simulink model "ssc_lithium_cell_1RC"  (R2019b)
settings: Solver=ode15s  StartTime=0.0  StopTime=40000  MaxStep=60  RelTol=1e-3  EnableMultiTasking=on
PreLoadFcn:
  | ssc_lithium_cell_1RC_ini
undefined symbols (not defined in the file): Battery, sigbuilder_block
libraries: fl_lib x8, nesl_utility x6, ee_lib x1
Description:
  | Lithium Battery Cell - One RC-Branch Equivalent Circuit
  | 
  | This example shows how to model a lithium cell using the Simscape(TM)
  | language to implement the elements of an equivalent circuit model
  | with one RC branch. For the defining equations and their validation,
  | see T. Huria, M. Ceraolo, J. Gazzarri, R. Jackey. "High Fidelity Electrical
  | Model with Thermal Dependence for Characterization and Simulation of
  | High Power Lithium Battery Cells," IEEE International Electric Vehicle
  | Conference, March 2012.
  | 
  | A simple thermal model is used to model battery temperature. It is
  | assumed that cooling is primarily via convection, and that heating is
  | primarily from internal resistance. A battery pack can be modeled by
  | connecting multiple copies of the battery cell block in series.
  | 
  | 
  | 
  | Copyright 2008-2012 The MathWorks, Inc.
settings Model: Creator=MathWorks  LastModifiedBy=cpatel
settings DataIOCC: LimitDataPoints=on  SaveFormat=Array  SignalLoggingSaveFormat=ModelDataLogs  SaveOutput=off  SaveTime=off
settings OptimizationCC: ExpressionDepthLimit=2147483647  LifeSpan=inf
settings DebuggingCC: StateNameClashWarn=warning  SFUnexpectedBacktrackingDiag=warning  SFNoUnconditionalDefaultTransitionDiag=warning  SFExecutionAtInitializationDiag=none  ArithmeticOperatorsInVariantConditions=warning
settings HardwareCC: ProdBitPerPointer=32  ProdBitPerSizeT=32  ProdBitPerPtrDiffT=32  ProdLargestAtomicFloat=None  ProdIntDivRoundTo=Undefined  ProdEndianess=Unspecified  ProdWordSize=32  ProdHWDeviceType=32-bit Generic
settings ModelReferenceCC: PropagateSignalLabelsOutOfModel=off
settings SFSimCC: SimUseLocalCustomCode=off  CustomCodeUndefinedFunction=UseInterfaceOnly
settings RTWCC: RTWUseLocalCustomCode=off
settings CodeAppCC: StateflowObjectComments=on
settings GRTTargetCC: TargetLangStandard=C89/C90 (ANSI)  GeneratePreprocessorConditionals=Disable all  CombineOutputUpdateFcns=off  GRTInterface=on
settings ConfigComp: CovMetricSettings=dw  CovHtmlReporting=on  CovSaveCumulativeToWorkspaceVar=on  CovSaveSingleToWorkspaceVar=on  CovExternalEMLEnable=off
settings SimscapeCC: SimscapeNormalizeSystem=off

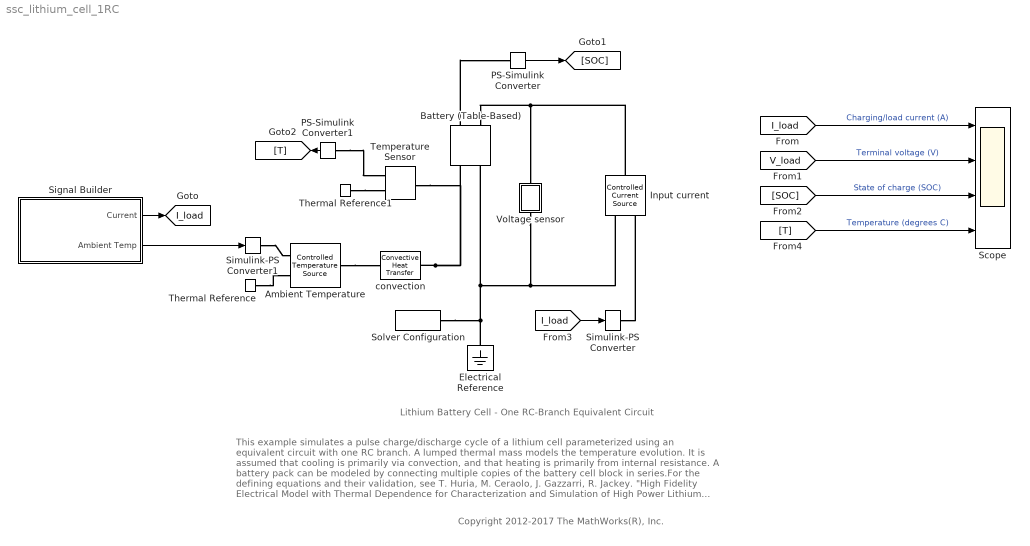
== system ssc_lithium_cell_1RC ==
  note: Lithium Battery Cell - One RC-Branch Equivalent Circuit
  note: This example simulates a pulse charge/discharge cycle of a lithium cell parameterized using an equivalent circuit with one RC branch. A lumped thermal mass models the temperature evolution. It is assumed that cooling is primarily via convection, and that heating is primarily from internal resistance. A battery pack can be modeled by connecting multiple copies of the battery cell block in series.For the defining equations and their validation, see T. Huria, M. Ceraolo, J. Gazzarri, R. Jackey. "High Fidelity Electrical Model with Thermal Dependence for Characterization and Simulation of High Power Lithium Battery Cells," IEEE International Electric Vehicle Conference, March 2012.
  note: Copyright 2012-2017 The MathWorks(R), Inc.
  Ambient Temperature : fl_lib/Thermal/Thermal Sources/Controlled Temperature Source
      settings: SourceProductName=Simscape
  Battery (Table-Based) : ee_lib/Sources/Battery (Table-Based)  SOC_vec=Battery.SOC_LUT  T_dependence=ee.enum.temperature_dependence.yes  T_vec=Battery.Temperature_LUT K  V0_mat=Battery.Em_LUT V  V0_vec=[3.1, 3.27, 3.31, 3.5] V  R0_mat=Battery.R0_LUT Ohm  R0_vec=[.015, .017, .012, .013] Ohm  AH_vec=Battery.Capacity_LUT hr*A  AH=4.1 hr*A  prm_leak=1  Rleak_vec=[8000, 7000, 6000] Ohm  Rleak=7e3 Ohm  prm_dyn=2  R1_mat=Battery.R1_LUT Ohm  R1_vec=[.076, .022, .007, .043] Ohm  tau1_mat=Battery.R1_LUT.*Battery.C1_LUT s  tau1_vec=[148, 110, 27, 22] s  R2_mat=[.014, .382, .407; .028, .006, .007; .014, .007, .006; .333, .956, .912] Ohm  R2_vec=[.382, .006, .007, .956] Ohm  tau2_mat=[1, 44, 5644; 11, 24, 506; 2, 14, 330; 3310, 13419, 30216] s  tau2_vec=[44, 24, 14, 13419] s  R3_mat=[.014, .382, .407; .028, .006, .007; .014, .007, .006; .333, .956, .912] Ohm  R3_vec=[.382, .006, .007, .956] Ohm  tau3_mat=[1, 44, 5644; 11, 24, 506; 2, 14, 330; 3310, 13419, 30216] s  tau3_vec=[44, 24, 14, 13419] s  R4_mat=[.014, .382, .407; .028, .006, .007; .014, .007, .006; .333, .956, .912] Ohm  R4_vec=[.382, .006, .007, .956] Ohm  tau4_mat=[1, 44, 5644; 11, 24, 506; 2, 14, 330; 3310, 13419, 30216] s  tau4_vec=[44, 24, 14, 13419] s  R5_mat=[.014, .382, .407; .028, .006, .007; .014, .007, .006; .333, .956, .912] Ohm  R5_vec=[.382, .006, .007, .956] Ohm  tau5_mat=[1, 44, 5644; 11, 24, 506; 2, 14, 330; 3310, 13419, 30216] s  tau5_vec=[44, 24, 14, 13419] s  prm_fade=ee.enum.battery.prm_fade.equations  N0=100  dV0=0  dR0=0  dAH=0  dRleak=0  dR1=0  dR2=0  dR3=0  dR4=0  dR5=0  N0vec=[100, 200, 300]  Tfadevec=[298.15, 323.15] K  dV0vec=[0, 0, 0]  dR0vec=[0, 0, 0]  dAHvec=[0, 0, 0]  dRleakvec=[0, 0, 0]  dR1vec=[0, 0, 0]  dR2vec=[0, 0, 0]  dR3vec=[0, 0, 0]  dR4vec=[0, 0, 0]  dR5vec=[0, 0, 0]  dV0mat=[0, 0; 0, 0; 0, 0]  dR0mat=[0, 0; 0, 0; 0, 0]  dAHmat=[0, 0; 0, 0; 0, 0]  dRleakmat=[0, 0; 0, 0; 0, 0]  dR1mat=[0, 0; 0, 0; 0, 0]  dR2mat=[0, 0; 0, 0; 0, 0]  dR3mat=[0, 0; 0, 0; 0, 0]  dR4mat=[0, 0; 0, 0; 0, 0]  dR5mat=[0, 0; 0, 0; 0, 0]  temperature=Battery.T_init K  i_specify=off  i_priority=None  i=0 A  i_nominal_specify=off  i_nominal_unit=A  i_nominal_value=1  v_specify=off  v_priority=None  v=0 V  v_nominal_specify=off  v_nominal_unit=V  v_nominal_value=1  stateOfCharge_specify=on  stateOfCharge_priority=High  stateOfCharge=(Battery.Capacity_LUT(2) - Battery.Qe_init)/Battery.Capacity_LUT(2)  stateOfCharge_nominal_specify=off  stateOfCharge_nominal_unit=1  stateOfCharge_nominal_value=1  num_cycles_specify=off  num_cycles_priority=High  num_cycles=0  num_cycles_nominal_specify=off  num_cycles_nominal_unit=1  num_cycles_nominal_value=1  thermal_mass=Battery.cell_Cp_heat*Battery.cell_mass J/K  temperature_specify=on  temperature_priority=High  temperature_nominal_specify=off  temperature_nominal_unit=K  temperature_nominal_value=1
      settings: SourceProductName=Simscape Electrical  SourceProductBaseCode=PS  InternalSimscapePortConfiguration="{\"Bottom\":[],\"Left\":[{\"id\":\"p\",\"label\":\"+\",\"type\":\"foundation.electrical.electrical\"},{\"id\":\"soc\",\"label\":\"SOC\",\"type\":\"output\"}],\"Right\":[{\"id\":\"n\",\"label\":\"-\",\"type\":\"foundation.electrical.electrical\"},{\"id\":\"H\",\"label\":\"H\",\"type\":\"foundation.thermal.thermal\"}],\"Top\":[]}"
  Electrical Reference : fl_lib/Electrical/Electrical Elements/Electrical Reference
  Input current : fl_lib/Electrical/Electrical Sources/Controlled Current Source
  PS-Simulink Converter : nesl_utility/PS-Simulink Converter  PhysicalDomain=network_engine_domain  SubClassName=ps_output  LeftPortType=input  RightPortType=output  PseudoPeriodic=off  Frequencies=[]  Unit=1  AffineConversion=off
  PS-Simulink Converter1 : nesl_utility/PS-Simulink Converter  PhysicalDomain=network_engine_domain  SubClassName=ps_output  LeftPortType=input  RightPortType=output  PseudoPeriodic=off  Frequencies=[]  Unit=K  AffineConversion=off
  Scope : Scope  NumInputPorts=4
  Signal Builder : Subsystem  Tag=STV Subsys  LoadFcn=sigbuilder_block('load');  StartFcn=sigbuilder_block('start');  StopFcn=sigbuilder_block('stop');  ClipboardFcn=sigbuilder_block('clipboard');  mask(Sigbuilder block){tuvar=[0:10]}
      mask help: Simulink:masks:SigbuilderBlock_MD
      mask init:
      | if ~strcmp(get_param(bdroot(gcbh),'SimulationStatus'),'stopped') tuvar = sigbuilder_block('maskInit'); end
      settings: CopyFcn=sigbuilder_block('copy');  DeleteFcn=sigbuilder_block('delete');  ModelCloseFcn=sigbuilder_block('modelClose');  PreSaveFcn=sigbuilder_block('preSave');  PauseFcn=sigbuilder_block('pause');  ContinueFcn=sigbuilder_block('continue');  NameChangeFcn=sigbuilder_block('namechange');  OpenFcn=sigbuilder_block('open',[33.75 101.25 755.25 399.75 ]);  CloseFcn=sigbuilder_block('close');
      mask Display: plot(0, 0, 100, 100,[2, 2, 32, 32, 2], [68, 8, 8, 68, 68],[32, 2], [38, 38], [32, 19, 2],[53, 60, 44], [32, 17, 17, 2],[16, 16, 31, 31]);txt = getActiveGroup(gcbh);text(2, 100, txt,'verticalAlignment', 'top');
  Simulink-PS Converter : nesl_utility/Simulink-PS Converter  PhysicalDomain=network_engine_domain  SubClassName=ps_input  LeftPortType=input  RightPortType=output  PseudoPeriodic=off  Frequencies=[]  NoiseDistribution=none  NoiseParameters=[]  Unit=A  AffineConversion=off  FilteringAndDerivatives=zero  SimscapeFilterOrder=1  InputFilterTimeConstant=.001  UdotUserProvided=1
  Simulink-PS Converter1 : nesl_utility/Simulink-PS Converter  PhysicalDomain=network_engine_domain  SubClassName=ps_input  LeftPortType=input  RightPortType=output  PseudoPeriodic=off  Frequencies=[]  NoiseDistribution=none  NoiseParameters=[]  Unit=degC  AffineConversion=on  FilteringAndDerivatives=zero  SimscapeFilterOrder=1  InputFilterTimeConstant=.001  UdotUserProvided=1
  Solver Configuration : nesl_utility/Solver Configuration  PhysicalDomain=network_engine_domain  SubClassName=solver  LeftPortType=input  RightPortType=generic  Tones=[]  Harmonics=[]  SimulateNoise=off  Profile=off  UseLocalSampling=off  EnableSwitchedLinearOptims=on  FrequencyDomain=off  UseCCode=off  RelTol=0.001  AbsTol=1e-06  MinStep=1e-09  ToWorkspace=off  RevertToSquareIcSolve=off  NumHomotopyIterations=100  PhasorMode=off  PhasorModeNumHarmonics=1  DoDC=off  ResidualTolerance=1e-9  UseLocalSolver=off  LocalSolverChoice=NE_BACKWARD_EULER_ADVANCER  LocalSolverSampleTime=1  DoFixedCost=off  MaxNonlinIter=3  MaxModeIter=2  LinearAlgebra=Sparse  EquationFormulation=NE_TIME_EF  DelaysMemoryBudget=1024  AutomaticFiltering=on  FilteringTimeConstant=0.001  PartitionStorageMethod=AS_NEEDED  PartitionMemoryBudget=1024  PartitionMethod=FAST
  Temperature Sensor : fl_lib/Thermal/Thermal Sensors/Temperature Sensor
  Thermal Reference : fl_lib/Thermal/Thermal Elements/Thermal Reference
  Thermal Reference1 : fl_lib/Thermal/Thermal Elements/Thermal Reference
  Voltage sensor : Subsystem
  convection : fl_lib/Thermal/Thermal Elements/Convective Heat Transfer  area=cell_area m^2  heat_tr_coeff=h_conv W/(m^2 * K)  T_specify=off  T_priority=None  T=0 K  T_nominal_specify=off  T_nominal_unit=K  T_nominal_value=1  Q_specify=off  Q_priority=None  Q=0 J/s  Q_nominal_specify=off  Q_nominal_unit=J/s  Q_nominal_value=1
  tag scope: I_load=global
  wires:
  [SOC] -> Scope/3  "State of charge (SOC)"
  [T] -> Scope/4  "Temperature (degrees C)"
  [I_load] -> Scope/1  "Charging/load current (A)"
  [V_load] -> Scope/2  "Terminal voltage (V)"
  Signal Builder/2(Ambient Temp) -> Simulink-PS Converter1/1
  Signal Builder/1(Current) -> [I_load]
  PS-Simulink Converter/1 -> [SOC]
  [I_load] -> Simulink-PS Converter/1
  PS-Simulink Converter1/1 -> [T]
  connections:
  Electrical Reference/LConn1 -- Solver Configuration/RConn1 -- Voltage sensor/RConn1 -- Input current/RConn2 -- Battery (Table-Based)/RConn1
  Input current/LConn1 -- Battery (Table-Based)/LConn1 -- Voltage sensor/LConn1
  Thermal Reference/LConn1 -- Ambient Temperature/RConn2
  Ambient Temperature/LConn1 -- convection/LConn1
  convection/RConn1 -- Temperature Sensor/LConn1 -- Battery (Table-Based)/RConn2
  Simulink-PS Converter/RConn1 -- Input current/RConn1
  Simulink-PS Converter1/RConn1 -- Ambient Temperature/RConn1
  Battery (Table-Based)/LConn2 -- PS-Simulink Converter/LConn1
  Thermal Reference1/LConn1 -- Temperature Sensor/RConn1
  PS-Simulink Converter1/LConn1 -- Temperature Sensor/RConn2

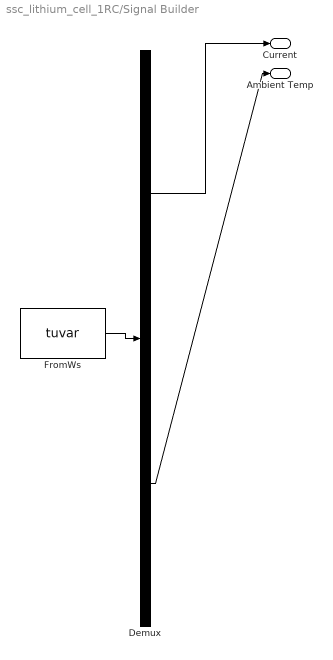
== system ssc_lithium_cell_1RC/Signal Builder ==
  Demux : Demux  Tag=STV Demux  Outputs=2
  FromWs : FromWorkspace  Tag=STV FromWs  VariableName=tuvar  SampleTime=0
      SigBuilderData=|
      | common.afterFinalStr = 'Extrapolate'
      | common.sampleTime = 0
      | dataSet(1).timeRange = [0 40000]
      | dataSet(1).name = 'Pulse'
      | dataSet(2).timeRange = [0 40000]
      | dataSet(2).name = 'Constant'
      | sbobj.Name = 'Signal Builder'
      | sbobj.Groups(1).Name = 'Pulse'
      | sbobj.Groups(1).Signals(1).Name = 'Current'
      | sbobj.Groups(1).Signals(1).XData = [0 300 300 2100 2100 3600 3600 3960 3960 7200 7200 7560 7560 10800 10800 11160 11160 14400 14400 14760 14760 18000 18000 18360 18360 21600 21600 21960 21960 25200 25200 25560 25560 28800 28800 29160 29160 32400 32400 32760 32760 36000 36000 36360 36360 40000]
      | sbobj.Groups(1).Signals(1).YData = [0 0 31.5 31.5 0 0 -27.625 -27.625 0 0 -27.625 -27.625 0 0 -27.625 -27.625 0 0 -27.625 -27.625 0 0 -27.625 -27.625 0 0 -27.625 -27.625 0 0 -27.625 -27.625 0 0 -27.625 -27.625 0 0 -27.625 -27.625 0 0 -27.625 -27.625 0 0]
      | sbobj.Groups(1).Signals(2).Name = 'Ambient Temp'
      | sbobj.Groups(1).Signals(2).XData = [0 300 2100 3600 3960 7200 7560 10800 11160 14400 14760 18000 18360 21600 21960 25200 25560 28800 29160 32400 32760 36000 36360 40000]
      | sbobj.Groups(1).Signals(2).YData = [20 20 20 20 20 20 20 20 20 20 20 20 20 20 20 20 20 20 20 20 20 20 20 20]
      | sbobj.Groups(1).TimeRange = [0 40000]
      | sbobj.Groups(2).Name = 'Constant'
      | sbobj.Groups(2).Signals(1).Name = 'Current'
      | sbobj.Groups(2).Signals(1).XData = [0 360 360 9100 9100 11800 11800 28200 33800 40000]
      | sbobj.Groups(2).Signals(1).YData = [0 0 -5 -5 0 0 5 5 0 0]
      | sbobj.Groups(2).Signals(2).Name = 'Ambient Temp'
      | sbobj.Groups(2).Signals(2).XData = [0 360 360 9100 9100 11800 11800 28200 33800 40000]
      | sbobj.Groups(2).Signals(2).YData = [20 20.09 20.09 22.275 22.275 22.95 22.95 27.05 28.45 30]
      | sbobj.Groups(2).TimeRange = [0 40000]
  Current : Outport  VectorParamsAs1DForOutWhenUnconnected=off
  Ambient Temp : Outport  Tag=STV Outport  Port=2  VectorParamsAs1DForOutWhenUnconnected=off
  wires:
  Demux/1 -> Current/1
  FromWs/1 -> Demux/1
  Demux/2 -> Ambient Temp/1

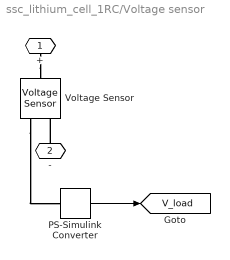
== system ssc_lithium_cell_1RC/Voltage sensor ==
  PS-Simulink Converter : nesl_utility/PS-Simulink Converter  PhysicalDomain=network_engine_domain  SubClassName=ps_output  LeftPortType=input  RightPortType=output  PseudoPeriodic=off  Frequencies=[]  Unit=V  AffineConversion=off
  Voltage Sensor : fl_lib/Electrical/Electrical Sensors/Voltage Sensor
  + : PMIOPort  Side=Left
  - : PMIOPort  Port=2  Side=Right
  tag scope: V_load=global
  wires:
  PS-Simulink Converter/1 -> [V_load]
  connections:
  Voltage Sensor/RConn1 -- PS-Simulink Converter/LConn1
  +/RConn1 -- Voltage Sensor/LConn1
  -/RConn1 -- Voltage Sensor/RConn2
